simulink model "CLSfixed"  (R2024b)
settings: Solver=FixedStepAuto  StartTime=0.0  StopTime=3000  FixedStep=stepsize  RelTol=1e-3
undefined symbols (not defined in the file or in its folder): AVI, cfg_length, LRI, pNode_length, pPath_length, PVARP, stepsize, URI, VRP
libraries: Libs_unified x311
(part 1 of 4)
settings Model: SimulationMode=accelerator  NumberOfSteps=8000  Creator=wai484  LastModifiedBy=ball907
settings SolverCC: AlgebraicLoopSolver=TrustRegion
settings DataIOCC: ReturnWorkspaceOutputs=off
settings DebuggingCC: UnconnectedInputMsg=warning  UnconnectedOutputMsg=warning  UnconnectedLineMsg=warning  ArithmeticOperatorsInVariantConditions=warning
settings ModelReferenceCC: EnableRefExpFcnMdlSchedulingChecks=on
settings SFSimCC: SimUseLocalCustomCode=off  CustomCodeUndefinedFunction=UseInterfaceOnly
settings RTWCC: RTWUseLocalCustomCode=off  BuildConfiguration=Faster Runs  GPUComputeCapability=3.5
settings CodeAppCC: StateflowObjectComments=on
settings GRTTargetCC: OptimizeReductions=on

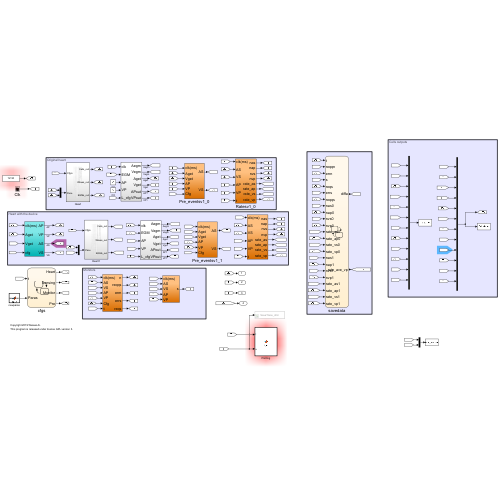
[thumbnail: Simulink's stored preview of the top-level diagram]
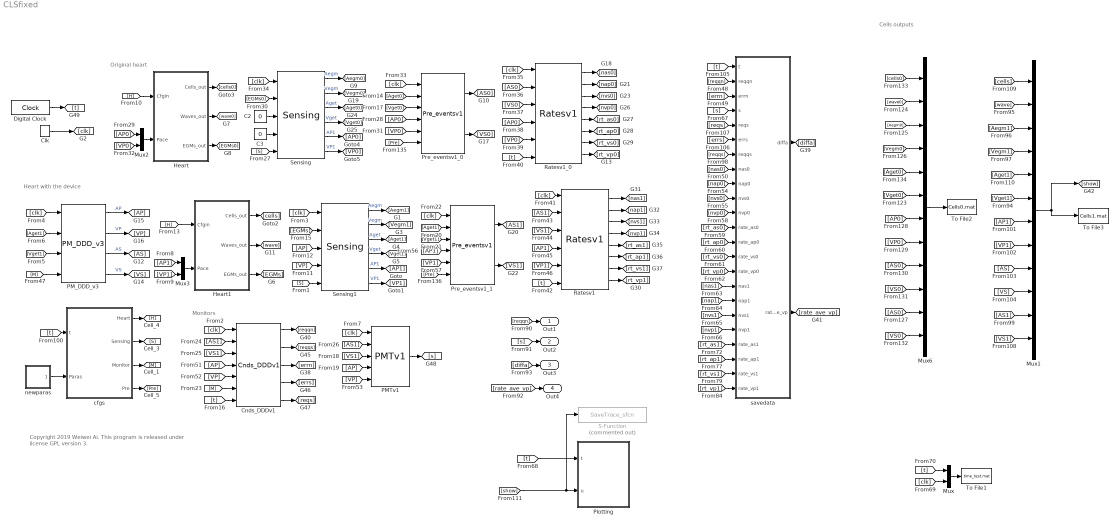
== system CLSfixed ==
  note: Heart with the device
  note: Original heart
  note: Monitors
  note: Copyright 2019 Weiwei Ai.
      | This program is released under license GPL version 3.
  note: Cells outputs
  C2 : Constant  Value=0
  C3 : Constant  Value=0
  Clk : DiscretePulseGenerator  PulseType=Time based  Period=1  PulseWidth=1/stepsize
  Cnds_DDDv1 : Libs_unified/Cnds_DDDv1  SystemSampleTime=-1  VariantActivationTime=update diagram  AllowFlexibleInterface=on  Latency=0  AutoFrameSizeCalculation=off
  Digital Clock : DigitalClock  SampleTime=stepsize
  Heart : Subsystem
  Heart1 : Subsystem
  Mux : Mux  Inputs=2
  Mux1 : Mux  Inputs=12
  Mux2 : Mux  Inputs=2
  Mux3 : Mux  Inputs=2
  Mux6 : Mux  Inputs=12
  PMTv1 : Libs_unified/PMTv1  SystemSampleTime=-1  VariantActivationTime=update diagram  AllowFlexibleInterface=on  Latency=0  AutoFrameSizeCalculation=off
  PM_DDD_v3 : Libs_unified/PM_DDD_v3  SystemSampleTime=-1  VariantActivationTime=update diagram  AllowFlexibleInterface=on  Latency=0  AutoFrameSizeCalculation=off
  Plotting : MATLAB Function  TreatAsAtomicUnit=on  SystemSampleTime=stepsize*5
  Pre_eventsv1_0 : Libs_unified/Pre_eventsv1  SystemSampleTime=-1  VariantActivationTime=update diagram  AllowFlexibleInterface=on  Latency=0  AutoFrameSizeCalculation=off
  Pre_eventsv1_1 : Libs_unified/Pre_eventsv1  SystemSampleTime=-1  VariantActivationTime=update diagram  AllowFlexibleInterface=on  Latency=0  AutoFrameSizeCalculation=off
  Ratesv1 : Libs_unified/Ratesv1  SystemSampleTime=-1  VariantActivationTime=update diagram  AllowFlexibleInterface=on  Latency=0  AutoFrameSizeCalculation=off
  Ratesv1_0 : Libs_unified/Ratesv1  SystemSampleTime=-1  VariantActivationTime=update diagram  AllowFlexibleInterface=on  Latency=0  AutoFrameSizeCalculation=off
  S-Function : S-Function  Commented=on  FunctionName=SaveTrace_sfcn  Parameters=1  SFunctionDeploymentMode=off  EnableBusSupport=off
  Sensing : Libs_unified/Sensing  SystemSampleTime=-1  VariantActivationTime=update diagram  AllowFlexibleInterface=on  Latency=0  AutoFrameSizeCalculation=off
  Sensing1 : Libs_unified/Sensing  SystemSampleTime=-1  VariantActivationTime=update diagram  AllowFlexibleInterface=on  Latency=0  AutoFrameSizeCalculation=off
  To File1 : ToFile  Filename=time_test.mat  MatrixName=digital_clock
      settings: Decimation=2
  To File2 : ToFile  Filename=Cells0.mat  MatrixName=cells
      settings: Decimation=2
  To File3 : ToFile  Filename=Cells1.mat  MatrixName=cells
      settings: Decimation=2
  cfgs : Stateflow chart  TreatAsAtomicUnit=on
  newparas : MATLAB Function  TreatAsAtomicUnit=on
  savedata : Stateflow chart  TreatAsAtomicUnit=on
  Out1 : Outport
  Out2 : Outport  Port=2
  Out3 : Outport  Port=3
  Out4 : Outport  Port=4
  wires:
  [M] -> PM_DDD_v3/4
  Clk/1 -> [clk]
  [clk] -> PM_DDD_v3/1
  [Aget1] -> PM_DDD_v3/2
  [Vget1] -> PM_DDD_v3/3
  Heart1/1(Cells_out) -> [cells]
  Heart1/2(Waves_out) -> [wave]
  Heart1/3(EGMs_out) -> [EGMs]
  cfgs/1(Heart) -> [H]
  cfgs/2(Sensing) -> [S]
  PM_DDD_v3/1 -> [AP]  "AP"
  PM_DDD_v3/2 -> [VP]  "VP"
  PM_DDD_v3/3 -> [AS]  "AS"
  PM_DDD_v3/4 -> [VS]  "VS"
  [AP1] -> Mux3/1
  [VP1] -> Mux3/2
  Sensing1/1 -> [Aegm1]  "Aegm"
  Sensing1/2 -> [Vegm1]  "Vegm"
  Sensing1/3 -> [Aget1]  "Aget"
  Sensing1/4 -> [Vget1]  "Vget"
  Sensing1/5 -> [AP1]  "AP1"
  Sensing1/6 -> [VP1]  "VP1"
  [clk] -> Pre_eventsv1_1/1
  [Aget1] -> Pre_eventsv1_1/2
  [Vget1] -> Pre_eventsv1_1/3
  [AP1] -> Pre_eventsv1_1/4
  [VP1] -> Pre_eventsv1_1/5
  [Pre] -> Pre_eventsv1_1/6
  Pre_eventsv1_1/1 -> [AS1]
  Pre_eventsv1_1/2 -> [VS1]
  cfgs/3(Monitor) -> [M]
  newparas/1(newparas) -> cfgs/2(Paras)
  [H] -> Heart1/1(Cfgin)
  Mux3/1 -> Heart1/2(Pace)
  Heart/1(Cells_out) -> [cells0]
  Heart/2(Waves_out) -> [wave0]
  Heart/3(EGMs_out) -> [EGMs0]
  [AP0] -> Mux2/1
  [H] -> Heart/1(Cfgin)
  Mux2/1 -> Heart/2(Pace)
  Sensing/1 -> [Aegm0]  "Aegm"
  Sensing/2 -> [Vegm0]  "Vegm"
  Sensing/3 -> [Aget0]  "Aget"
  Sensing/4 -> [Vget0]  "Vget"
  Sensing/5 -> [AP0]  "AP1"
  Sensing/6 -> [VP0]  "VP1"
  [clk] -> Pre_eventsv1_0/1
  [Aget0] -> Pre_eventsv1_0/2
  [Vget0] -> Pre_eventsv1_0/3
  [AP0] -> Pre_eventsv1_0/4
  [Pre] -> Pre_eventsv1_0/6
  Pre_eventsv1_0/1 -> [AS0]
  Pre_eventsv1_0/2 -> [VS0]
  [VP0] -> Pre_eventsv1_0/5
  [VP0] -> Mux2/2
  [clk] -> Sensing/1
  [S] -> Sensing/5
  C3/1 -> Sensing/4
  C2/1 -> Sensing/3
  [EGMs0] -> Sensing/2
  [clk] -> Sensing1/1
  [EGMs] -> Sensing1/2
  [AP] -> Sensing1/3
  [VP] -> Sensing1/4
  [S] -> Sensing1/5
  Digital Clock/1 -> [t]
  [t] -> cfgs/1(t)
  cfgs/4(Pre) -> [Pre]
  [clk] -> Ratesv1_0/1
  [AS0] -> Ratesv1_0/2
  [VS0] -> Ratesv1_0/3
  [AP0] -> Ratesv1_0/4
  [VP0] -> Ratesv1_0/5
  [t] -> Ratesv1_0/6
  Ratesv1_0/1 -> [nas0]
  Ratesv1_0/2 -> [nap0]
  Ratesv1_0/3 -> [nvs0]
  Ratesv1_0/4 -> [nvp0]
  Ratesv1_0/5 -> [rt_as0]
  Ratesv1_0/6 -> [rt_ap0]
  Ratesv1_0/7 -> [rt_vs0]
  Ratesv1_0/8 -> [rt_vp0]
  [clk] -> Ratesv1/1
  [t] -> Ratesv1/6
  Ratesv1/1 -> [nas1]
  Ratesv1/2 -> [nap1]
  Ratesv1/3 -> [nvs1]
  Ratesv1/4 -> [nvp1]
  Ratesv1/5 -> [rt_as1]
  Ratesv1/6 -> [rt_ap1]
  Ratesv1/7 -> [rt_vs1]
  Ratesv1/8 -> [rt_vp1]
  [AS1] -> Ratesv1/2
  [VS1] -> Ratesv1/3
  [AP1] -> Ratesv1/4
  [VP1] -> Ratesv1/5
  Cnds_DDDv1/1 -> [reqqn]
  Cnds_DDDv1/2 -> [reqqs]
  Cnds_DDDv1/5 -> [reqs]
  [AP] -> PMTv1/4
  [VP] -> PMTv1/5
  [AS1] -> Cnds_DDDv1/2
  [VS1] -> Cnds_DDDv1/3
  [AP] -> Cnds_DDDv1/4
  [VP] -> Cnds_DDDv1/5
  [M] -> Cnds_DDDv1/6
  [t] -> Cnds_DDDv1/7
  Cnds_DDDv1/4 -> [errs]
  Cnds_DDDv1/3 -> [errn]
  [clk] -> Cnds_DDDv1/1
  PMTv1/1 -> [s]
  [VS1] -> PMTv1/3
  [AS1] -> PMTv1/2
  [clk] -> PMTv1/1
  [t] -> savedata/1(t)
  [reqqn] -> savedata/2(reqqn)
  [errn] -> savedata/3(errn)
  [s] -> savedata/4(s)
  [errs] -> savedata/6(errs)
  [reqs] -> savedata/5(reqs)
  [reqqs] -> savedata/7(reqqs)
  [nas0] -> savedata/8(nas0)
  [nap0] -> savedata/9(nap0)
  [nvs0] -> savedata/10(nvs0)
  [nvp0] -> savedata/11(nvp0)
  [rt_as0] -> savedata/12(rate_as0)
  [rt_ap0] -> savedata/13(rate_ap0)
  [rt_vs0] -> savedata/14(rate_vs0)
  [rt_vp0] -> savedata/15(rate_vp0)
  [nas1] -> savedata/16(nas1)
  [nap1] -> savedata/17(nap1)
  [nvs1] -> savedata/18(nvs1)
  [nvp1] -> savedata/19(nvp1)
  [rt_as1] -> savedata/20(rate_as1)
  [rt_ap1] -> savedata/21(rate_ap1)
  [rt_vs1] -> savedata/22(rate_vs1)
  [rt_vp1] -> savedata/23(rate_vp1)
  savedata/1(diffa) -> [diffa]
  savedata/2(rate_ave_vp) -> [rate_ave_vp]
  [reqqn] -> Out1/1
  [s] -> Out2/1
  [diffa] -> Out3/1
  [rate_ave_vp] -> Out4/1
  [wave0] -> Mux6/2
  [Aegm0] -> Mux6/3
  [Vegm0] -> Mux6/4
  [cells0] -> Mux6/1
  [Aget0] -> Mux6/5
  [Vget0] -> Mux6/6
  [AP0] -> Mux6/7
  [VP0] -> Mux6/8
  [AS0] -> Mux6/9
  [VS0] -> Mux6/10
  [AS0] -> Mux6/11
  [VS0] -> Mux6/12
  [wave] -> Mux1/2
  [Aegm1] -> Mux1/3
  [Vegm1] -> Mux1/4
  [cells] -> Mux1/1
  [Aget1] -> Mux1/5
  [Vget1] -> Mux1/6
  [AP1] -> Mux1/7
  [VP1] -> Mux1/8
  [AS] -> Mux1/9
  [VS] -> Mux1/10
  [AS1] -> Mux1/11
  [VS1] -> Mux1/12
  Mux6/1 -> To File2/1
  Mux1/1 -> To File3/1, [show]
  [show] -> S-Function/1, Plotting/2(u)
  [t] -> Plotting/1(t)
  [t] -> Mux/1
  [clk] -> Mux/2
  Mux/1 -> To File1/1
